simulink model "MuscleSpindleTest"  (Simulink 8.1)
settings: Solver=ode3  StartTime=0.0  StopTime=3.3  FixedStep=1e-3  MinStep=1e-12  RelTol=1e-4
libraries: simulink x1
settings Model: Creator=oli  LastModifiedBy=mitkof6
settings DebuggingCC: FcnCallInpInsideContextMsg=EnableAllAsWarning
settings GRTTargetCC: CombineOutputUpdateFcns=on  GRTInterface=off

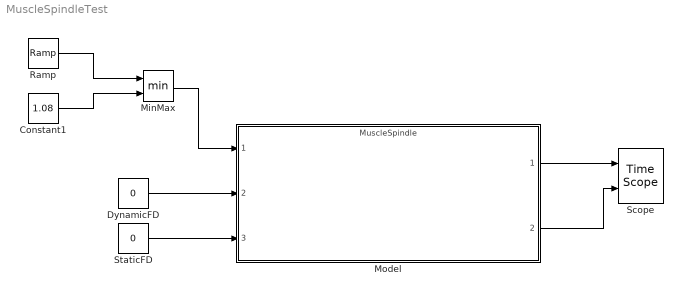
== system MuscleSpindleTest ==
  Constant1 : Constant  Value=1.08
  DynamicFD : Constant  Value=0
  MinMax : MinMax  Inputs=2
  Model : ModelReference  ModelNameDialog=MuscleSpindle  SimulationMode=Normal  ModelReferenceVersion=1.477  CopyOfModelName=MuscleSpindle  DefaultDataLogging=on
  Ramp : simulink/Sources/Ramp  slope=0.66  start=1  X0=0.95
  Scope : TimeScope  NumInputPorts=2  DefaultConfigurationName=spbscopes.TimeScopeBlockCfg
      settings: CopyFcn=scopeextensions.ScopeBlock.callback(gcbh, 'onBlockCopy', gcbh);  DeleteFcn=scopeextensions.ScopeBlock.callback(gcbh, 'onBlockDelete');  PreSaveFcn=scopeextensions.ScopeBlock.callback(gcbh, 'onModelSave');  NameChangeFcn=scopeextensions.ScopeBlock.callback(gcbh, 'onBlockRename');  OpenFcn=scopeextensions.SrcWiredSL.coreBlockCommand('Open',gcbh)  CloseFcn=scopeextensions.ScopeBlock.callback(gcbh, 'onBlockClose');  PreDeleteFcn=scopeextensions.ScopeBlock.callback(gcbh, 'onBlockPreDelete');
  StaticFD : Constant  Value=0
  wires:
  Ramp/1 -> MinMax/1
  Constant1/1 -> MinMax/2
  MinMax/1 -> Model/1
  DynamicFD/1 -> Model/2
  StaticFD/1 -> Model/3
  Model/2 -> Scope/2
  Model/1 -> Scope/1
